simulink model "prova1"  (R2019b)
settings: Solver=VariableStepAuto  StartTime=0.0  StopTime=50  RelTol=1e-3
libraries: simulink x1
settings Model: Creator=sugam  LastModifiedBy=sugam

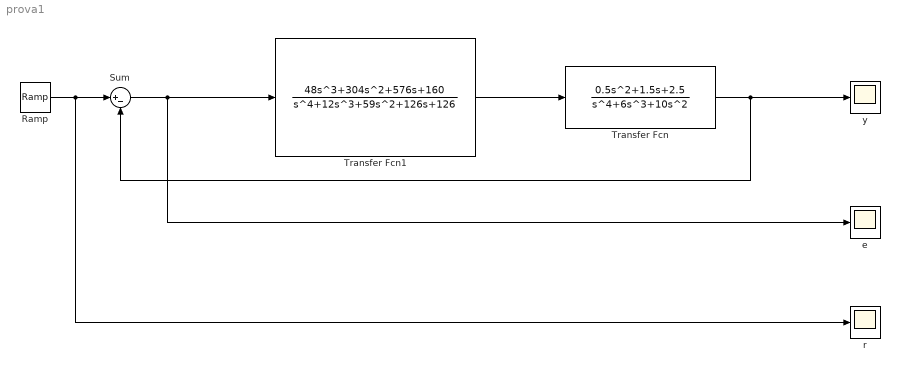
== system prova1 ==
  Ramp : simulink/Sources/Ramp  slope=1  start=0  InitialOutput=0
  Sum : Sum  Inputs=|+-
  Transfer Fcn : TransferFcn  Numerator=[0.5 1.5 2.5]  Denominator=[1 6 10 0 0]
  Transfer Fcn1 : TransferFcn  Numerator=[0 48 304 576 160]  Denominator=[1 12 59 126 126]
  e : Scope
  r : Scope
  y : Scope
  wires:
  Transfer Fcn/1 -> Sum/2, y/1
  Sum/1 -> e/1, Transfer Fcn1/1
  Ramp/1 -> r/1, Sum/1
  Transfer Fcn1/1 -> Transfer Fcn/1
